simulink model "ekf_model"  (R2019a)
settings: Solver=VariableStepAuto  StartTime=0.0  StopTime=15  RelTol=1e-3
libraries: simulink_extras x1
settings Model: Creator=phand  LastModifiedBy=phand

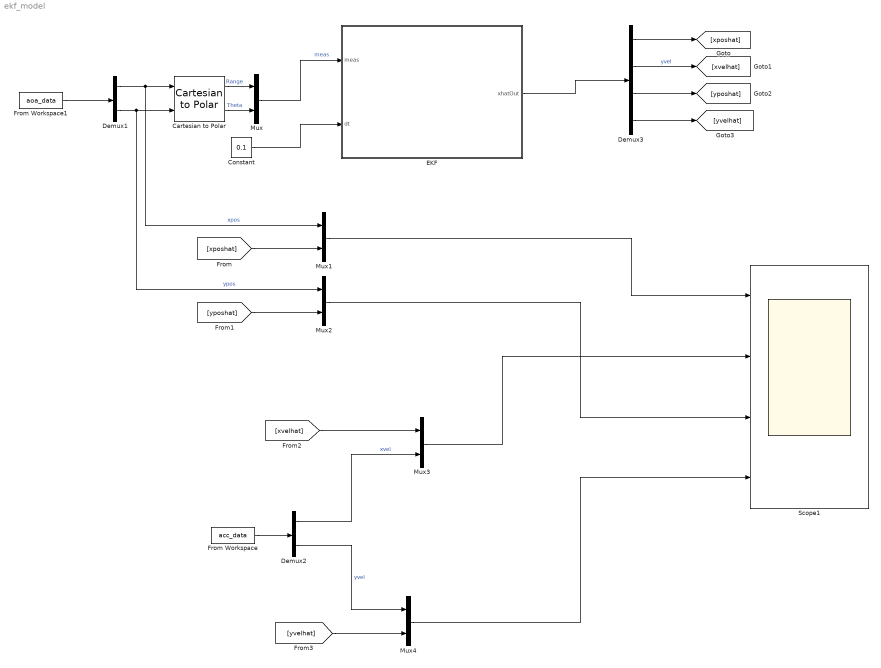
== system ekf_model ==
  Cartesian to Polar : simulink_extras/Transformations/Cartesian to Polar
      settings: SourceProductName=Simulink
  Constant : Constant  Value=0.1
  Demux1 : Demux  Outputs=2
  Demux2 : Demux  Outputs=2
  Demux3 : Demux
  "EKF " : MATLAB Function  TreatAsAtomicUnit=on
  From Workspace : FromWorkspace  VariableName=acc_data  SampleTime=0
  From Workspace1 : FromWorkspace  VariableName=aoa_data  SampleTime=0
  Mux{,1..4} (5 alike) : Mux  Inputs=2
  Scope1 : Scope  NumInputPorts=4
  wires:
  From Workspace1/1 -> Demux1/1
  Demux1/1 -> Mux1/1, Cartesian to Polar/1  "xpos"
  Demux1/2 -> Mux2/1, Cartesian to Polar/2  "ypos"
  Cartesian to Polar/1 -> Mux/1  "Range"
  Cartesian to Polar/2 -> Mux/2  "Theta"
  Demux3/4 -> [yvelhat]
  Demux3/3 -> [yposhat]
  Demux3/2 -> [xvelhat]  "yvel"
  Demux3/1 -> [xposhat]
  [xposhat] -> Mux1/2
  [yposhat] -> Mux2/2
  Mux1/1 -> Scope1/1
  From Workspace/1 -> Demux2/1
  [xvelhat] -> Mux3/1
  Demux2/1 -> Mux3/2  "xvel"
  [yvelhat] -> Mux4/2
  Demux2/2 -> Mux4/1  "yvel"
  Mux2/1 -> Scope1/3
  Mux3/1 -> Scope1/2
  Mux4/1 -> Scope1/4
  Mux/1 -> "EKF "/1(meas)  "meas"
  Constant/1 -> "EKF "/2(dt)
  "EKF "/1(xhatOut) -> Demux3/1

== matlab function ekf_model/EKF  ==
  data: meas input; xhatOut output; dt input
function xhatOut = EKF(meas, dt)
% This Embedded MATLAB Function implements an extended Kalman filter used
% for object tracking.
%
% The states of the process are given by
% x = [x_position; x_velocity; y_position; y_velocity];
%
% and the measurements are given by
% y = [range; bearing]
%
% where 
% range = sqrt(x_position^2 + y_position^2)
% bearing = atan2(y_position/x_position)

% Author: Phil Goddard (phil@goddardconsulting.ca)
% Date: Q2, 2011.

% Define storage for the variables that need to persist
% between time periods.
persistent P xhat Q R
if isempty(P)
    [xvel, yvel] = acc_init(35);
    %[xpos, ypos] = aoa_init(35);
    %[xinit, yinit] = acc_init(35);
    %[xposinit, yposinit] = aoa_init(35);
    xpos = 3;
    %xvel = 3.5;
    ypos = 4.2;
    %yvel = 1.2;
    
    % First time through the code so do some initialization
    xhat = [xpos; xvel; ypos; yvel];
    %xhat = [-900;80;950;20];
    P = zeros(4,4);
    Q =  diag([0 .1 0 .1]);
    R =  diag([50^2 0.005^2]);
end
% Calculate the Jacobians for the state and measurement equations
F = [1 dt 0 0;0 1 0 0;0 0 1 dt;0 0 0 1];
rangeHat = sqrt(xhat(1)^2+xhat(3)^2);
bearingHat = atan2(xhat(3),xhat(1));
yhat = [rangeHat; bearingHat]; 
H = [cos(bearingHat) 0 sin(bearingHat) 0;
    -sin(bearingHat)/rangeHat 0 cos(bearingHat)/rangeHat 0];

% Propogate the state and covariance matrices
xhat = F*xhat;
P = F*P*F' + Q;

% Calculate the Kalman gain
K = P*H'/(H*P*H' + R);

% Calculate the measurement residual
resid = meas - yhat;

% Update the state and covariance estimates
xhat = xhat + K*resid;
P = (eye(size(K,1))-K*H)*P;

% Post the results
xhatOut = xhat;
